simulink model "MVDR_example_hdl_4x4_systolic"  (R2020a)
settings: Solver=FixedStepDiscrete  StartTime=0.0  StopTime=stoptime  RelTol=1e-3
InitFcn:
  | model_init
values from neighbouring files (symbols this model uses):
  BackSubstitutePrototype = fi(0, matrixdivbacksub_dt)    [model_init.m]
  matrixDivDelay = NumberOfCORDICIterations*10 + 86    [model_init.m]
  movavg_bitshift = nextpow2(sqrt(windowSize))    [model_init.m]
  mvdrPipelineDelay = covMatDelay+movAvgDelay+matrixDivDelay+normResponseDelay    [model_init.m]
  numArrayElements = 4    [model_init.m]
  NumberOfCORDICIterations = matrixdivin_dt.WordLength - 1    [model_init.m]
  srcAngles = [20 60]    [model_init.m]
  sv = step(steeringVector,fc,[scanAngle; 0])    [model_init.m]
  Ts = 1/fs    (= 7.8125e-09)    [model_init.m]
  windowSize = 1024    [model_init.m]
libraries: hdlsllib x249, simulink x44, commfilt2 x4, commrfcorlib x3, commsync2 x3, commrflib2 x2, commrandsrc3 x2, phasedtxrxlib x2, commdigbbndcpm2 x1, dspsolvers x1, embreciprocals x1, commdigbbndpm3 x1
(part 3 of 11)

== system MVDR_example_hdl_4x4_systolic/MVDR HDL/Compute Weight Vector/Matrix Left Divide/CORDIC/4x4 Complex CORDIC Matrix Left Divide/Q'B, R 4x4 Complex CORDIC Systolic Array/Complex Row Rotation with real pivots ==
  note: The pivots are real, so you don't need to
      | rotate the first elements to real, but you do
      | need to account for the delay in the parallel
      | elements that are rotating their first elements
      | to real.
  x : Inport
  y : Inport  Port=2
  u : Inport  Port=3
  v : Inport  Port=4
  validIn : Inport  Port=5
  validIn from rotate first element to real : Inport  Port=6
  Delay17 : Delay  DelayLength=1
  Delay18 : Delay  DelayLength=1
  Delay2 : Delay  DelayLength=1
  Inverse CORDIC Gain1 : Subsystem  TreatAsAtomicUnit=on  mask{NumberOfCORDICIterations=NumberOfCORDICIterations}
      mask prompts: NumberOfCORDICIterations "Number of CORDIC Iterations"
      mask Display: disp('1/An')
  Inverse CORDIC Gain2 : Subsystem  TreatAsAtomicUnit=on  mask{NumberOfCORDICIterations=NumberOfCORDICIterations}
      mask prompts: NumberOfCORDICIterations "Number of CORDIC Iterations"
      mask Display: disp('1/An')
  Inverse CORDIC Gain3 : Subsystem  TreatAsAtomicUnit=on  mask{NumberOfCORDICIterations=NumberOfCORDICIterations}
      mask prompts: NumberOfCORDICIterations "Number of CORDIC Iterations"
      mask Display: disp('1/An')
  Inverse CORDIC Gain4 : Subsystem  TreatAsAtomicUnit=on  mask{NumberOfCORDICIterations=NumberOfCORDICIterations}
      mask prompts: NumberOfCORDICIterations "Number of CORDIC Iterations"
      mask Display: disp('1/An')
  "Q'B, R Row Rotations - Complex" : Subsystem  TreatAsAtomicUnit=on  mask{NumberOfCORDICIterations=NumberOfCORDICIterations}
      mask prompts: NumberOfCORDICIterations "Number of CORDIC Iterations"
  QR 3rd and 4th Quadrant Compensation : MATLAB Function  TreatAsAtomicUnit=on
  Unit Delay Enabled Synchronous{,1..7,9..12} (12 alike) : hdlsllib/Discrete/Unit Delay Enabled Synchronous  InitialCondition=0.0  SampleTime=-1
      settings: SourceProductBaseCode=SL
  ValidIn to Ready Logic : Subsystem
  ValidIn to Ready Logic1 : Subsystem
  y = u(2:end) : MATLAB Function  TreatAsAtomicUnit=on
  x' : Outport  VectorParamsAs1DForOutWhenUnconnected=off
  y' : Outport  Port=2  VectorParamsAs1DForOutWhenUnconnected=off
  u' : Outport  Port=3  VectorParamsAs1DForOutWhenUnconnected=off
  v' : Outport  Port=4  VectorParamsAs1DForOutWhenUnconnected=off
  validOut : Outport  Port=5  VectorParamsAs1DForOutWhenUnconnected=off
  ready : Outport  Port=6  VectorParamsAs1DForOutWhenUnconnected=off
  wires:
  Inverse CORDIC Gain3/1(Out1) -> Unit Delay Enabled Synchronous4/1
  Inverse CORDIC Gain4/1(Out1) -> Unit Delay Enabled Synchronous7/1
  x/1 -> Unit Delay Enabled Synchronous3/1
  Unit Delay Enabled Synchronous3/1 -> Unit Delay Enabled Synchronous12/1
  y/1 -> Unit Delay Enabled Synchronous2/1
  u/1 -> Unit Delay Enabled Synchronous1/1
  Unit Delay Enabled Synchronous1/1 -> Unit Delay Enabled Synchronous10/1
  v/1 -> Unit Delay Enabled Synchronous/1
  Inverse CORDIC Gain2/1(Out1) -> Unit Delay Enabled Synchronous5/1
  "Q'B, R Row Rotations - Complex"/1(x_out) -> Inverse CORDIC Gain4/1(In1)
  "Q'B, R Row Rotations - Complex"/3(u_out) -> Inverse CORDIC Gain2/1(In1)
  "Q'B, R Row Rotations - Complex"/4(v_out) -> Inverse CORDIC Gain3/1(In1)
  Inverse CORDIC Gain1/1(Out1) -> Unit Delay Enabled Synchronous6/1
  y = u(2:end)/1(y) -> y'/1
  Unit Delay Enabled Synchronous2/1 -> Unit Delay Enabled Synchronous11/1
  Unit Delay Enabled Synchronous/1 -> Unit Delay Enabled Synchronous9/1
  "Q'B, R Row Rotations - Complex"/2(y_out) -> Inverse CORDIC Gain1/1(In1)
  Unit Delay Enabled Synchronous7/1 -> x'/1
  Unit Delay Enabled Synchronous6/1 -> y = u(2:end)/1(u)
  Unit Delay Enabled Synchronous5/1 -> u'/1
  Unit Delay Enabled Synchronous4/1 -> v'/1
  validIn from rotate first element to real/1 -> ValidIn to Ready Logic1/2(validIn), Delay2/1, Unit Delay Enabled Synchronous9/2, Unit Delay Enabled Synchronous10/2, Unit Delay Enabled Synchronous11/2, Unit Delay Enabled Synchronous12/2
  Delay17/1 -> validOut/1
  Delay18/1 -> ready/1
  "Q'B, R Row Rotations - Complex"/5(validOut) -> Delay17/1, Unit Delay Enabled Synchronous4/2, Unit Delay Enabled Synchronous5/2, Unit Delay Enabled Synchronous6/2, Unit Delay Enabled Synchronous7/2
  validIn/1 -> Unit Delay Enabled Synchronous/2, Unit Delay Enabled Synchronous1/2, Unit Delay Enabled Synchronous2/2, Unit Delay Enabled Synchronous3/2
  Unit Delay Enabled Synchronous12/1 -> QR 3rd and 4th Quadrant Compensation/1(x)
  Unit Delay Enabled Synchronous11/1 -> QR 3rd and 4th Quadrant Compensation/2(y)
  Unit Delay Enabled Synchronous10/1 -> QR 3rd and 4th Quadrant Compensation/3(u)
  Unit Delay Enabled Synchronous9/1 -> QR 3rd and 4th Quadrant Compensation/4(v)
  ValidIn to Ready Logic/1(readyOut) -> ValidIn to Ready Logic1/1(readyIn)
  ValidIn to Ready Logic1/1(readyOut) -> Delay18/1
  QR 3rd and 4th Quadrant Compensation/1(x_out) -> "Q'B, R Row Rotations - Complex"/1(x)
  QR 3rd and 4th Quadrant Compensation/2(y_out) -> "Q'B, R Row Rotations - Complex"/2(y)
  QR 3rd and 4th Quadrant Compensation/3(u_out) -> "Q'B, R Row Rotations - Complex"/3(u)
  QR 3rd and 4th Quadrant Compensation/4(v_out) -> "Q'B, R Row Rotations - Complex"/4(v)
  Delay2/1 -> "Q'B, R Row Rotations - Complex"/5(validIn), ValidIn to Ready Logic/2(validIn)
  "Q'B, R Row Rotations - Complex"/6(ready) -> ValidIn to Ready Logic/1(readyIn)

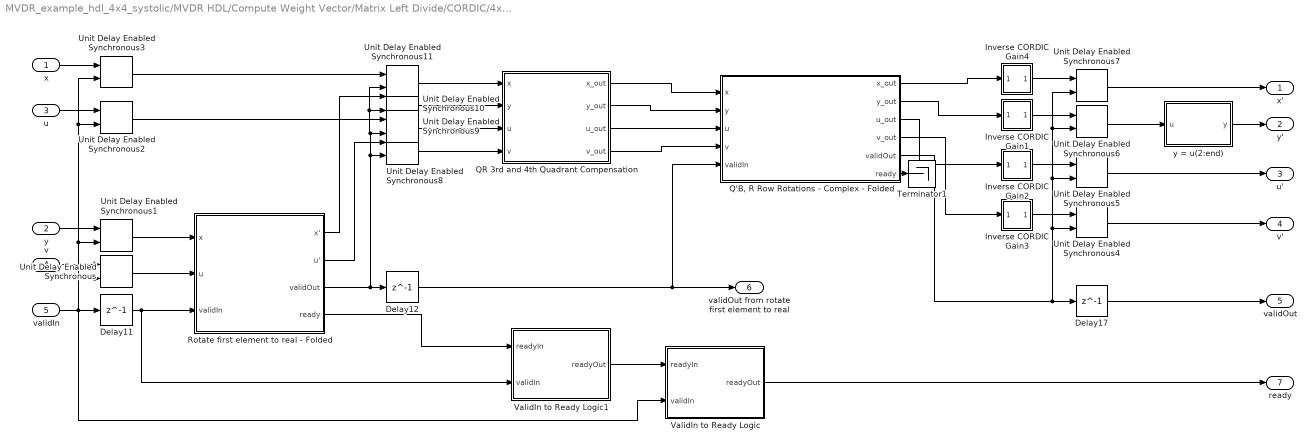
== system MVDR_example_hdl_4x4_systolic/MVDR HDL/Compute Weight Vector/Matrix Left Divide/CORDIC/4x4 Complex CORDIC Matrix Left Divide/Q'B, R 4x4 Complex CORDIC Systolic Array/Complex Row Rotation 1 ==
  x : Inport
  y : Inport  Port=2
  u : Inport  Port=3
  v : Inport  Port=4
  validIn : Inport  Port=5
  Delay11 : Delay  DelayLength=1
  Delay12 : Delay  DelayLength=1
  Delay17 : Delay  DelayLength=1
  Inverse CORDIC Gain1 : Subsystem  TreatAsAtomicUnit=on  mask{NumberOfCORDICIterations=NumberOfCORDICIterations}
      mask prompts: NumberOfCORDICIterations "Number of CORDIC Iterations"
      mask Display: disp('1/An')
  Inverse CORDIC Gain2 : Subsystem  TreatAsAtomicUnit=on  mask{NumberOfCORDICIterations=NumberOfCORDICIterations}
      mask prompts: NumberOfCORDICIterations "Number of CORDIC Iterations"
      mask Display: disp('1/An')
  Inverse CORDIC Gain3 : Subsystem  TreatAsAtomicUnit=on  mask{NumberOfCORDICIterations=NumberOfCORDICIterations}
      mask prompts: NumberOfCORDICIterations "Number of CORDIC Iterations"
      mask Display: disp('1/An')
  Inverse CORDIC Gain4 : Subsystem  TreatAsAtomicUnit=on  mask{NumberOfCORDICIterations=NumberOfCORDICIterations}
      mask prompts: NumberOfCORDICIterations "Number of CORDIC Iterations"
      mask Display: disp('1/An')
  "Q'B, R Row Rotations - Complex - Folded" : Subsystem  TreatAsAtomicUnit=on  mask{NumberOfCORDICIterations=NumberOfCORDICIterations}
      mask prompts: NumberOfCORDICIterations "Number of CORDIC Iterations"
  QR 3rd and 4th Quadrant Compensation : MATLAB Function  TreatAsAtomicUnit=on
  Rotate first element to real - Folded : Subsystem  TreatAsAtomicUnit=on  mask{NumberOfCORDICIterations=NumberOfCORDICIterations}
      mask prompts: NumberOfCORDICIterations "Number of CORDIC Iterations"
  Terminator1 : Terminator
  Unit Delay Enabled Synchronous{,1..11} (12 alike) : hdlsllib/Discrete/Unit Delay Enabled Synchronous  InitialCondition=0.0  SampleTime=-1
      settings: SourceProductBaseCode=SL
  ValidIn to Ready Logic : Subsystem
  ValidIn to Ready Logic1 : Subsystem
  y = u(2:end) : MATLAB Function  TreatAsAtomicUnit=on
  x' : Outport  VectorParamsAs1DForOutWhenUnconnected=off
  y' : Outport  Port=2  VectorParamsAs1DForOutWhenUnconnected=off
  u' : Outport  Port=3  VectorParamsAs1DForOutWhenUnconnected=off
  v' : Outport  Port=4  VectorParamsAs1DForOutWhenUnconnected=off
  validOut : Outport  Port=5  VectorParamsAs1DForOutWhenUnconnected=off
  validOut from rotate first element to real : Outport  Port=6  VectorParamsAs1DForOutWhenUnconnected=off
  ready : Outport  Port=7  VectorParamsAs1DForOutWhenUnconnected=off
  wires:
  "Q'B, R Row Rotations - Complex - Folded"/2(y_out) -> Inverse CORDIC Gain1/1(In1)
  "Q'B, R Row Rotations - Complex - Folded"/4(v_out) -> Inverse CORDIC Gain3/1(In1)
  "Q'B, R Row Rotations - Complex - Folded"/3(u_out) -> Inverse CORDIC Gain2/1(In1)
  ValidIn to Ready Logic/1(readyOut) -> ready/1
  x/1 -> Unit Delay Enabled Synchronous3/1
  ValidIn to Ready Logic1/1(readyOut) -> ValidIn to Ready Logic/1(readyIn)
  Inverse CORDIC Gain1/1(Out1) -> Unit Delay Enabled Synchronous6/1
  Unit Delay Enabled Synchronous4/1 -> v'/1
  Unit Delay Enabled Synchronous3/1 -> Unit Delay Enabled Synchronous11/1
  Rotate first element to real - Folded/4(ready) -> ValidIn to Ready Logic1/1(readyIn)
  Delay17/1 -> validOut/1
  Inverse CORDIC Gain2/1(Out1) -> Unit Delay Enabled Synchronous5/1
  Unit Delay Enabled Synchronous7/1 -> x'/1
  Delay12/1 -> validOut from rotate first element to real/1, "Q'B, R Row Rotations - Complex - Folded"/5(validIn)
  validIn/1 -> ValidIn to Ready Logic/2(validIn), Unit Delay Enabled Synchronous/2, Unit Delay Enabled Synchronous1/2, Unit Delay Enabled Synchronous2/2, Unit Delay Enabled Synchronous3/2, Delay11/1
  "Q'B, R Row Rotations - Complex - Folded"/6(ready) -> Terminator1/1
  v/1 -> Unit Delay Enabled Synchronous/1
  y/1 -> Unit Delay Enabled Synchronous1/1
  Unit Delay Enabled Synchronous5/1 -> u'/1
  "Q'B, R Row Rotations - Complex - Folded"/5(validOut) -> Delay17/1, Unit Delay Enabled Synchronous4/2, Unit Delay Enabled Synchronous5/2, Unit Delay Enabled Synchronous6/2, Unit Delay Enabled Synchronous7/2
  u/1 -> Unit Delay Enabled Synchronous2/1
  Unit Delay Enabled Synchronous6/1 -> y = u(2:end)/1(u)
  Inverse CORDIC Gain3/1(Out1) -> Unit Delay Enabled Synchronous4/1
  Unit Delay Enabled Synchronous2/1 -> Unit Delay Enabled Synchronous9/1
  Inverse CORDIC Gain4/1(Out1) -> Unit Delay Enabled Synchronous7/1
  "Q'B, R Row Rotations - Complex - Folded"/1(x_out) -> Inverse CORDIC Gain4/1(In1)
  Unit Delay Enabled Synchronous/1 -> Rotate first element to real - Folded/2(u)
  y = u(2:end)/1(y) -> y'/1
  Unit Delay Enabled Synchronous1/1 -> Rotate first element to real - Folded/1(x)
  Rotate first element to real - Folded/3(validOut) -> Unit Delay Enabled Synchronous10/2, Unit Delay Enabled Synchronous11/2, Unit Delay Enabled Synchronous9/2, Unit Delay Enabled Synchronous8/2, Delay12/1
  Delay11/1 -> ValidIn to Ready Logic1/2(validIn), Rotate first element to real - Folded/3(validIn)
  Rotate first element to real - Folded/1(x') -> Unit Delay Enabled Synchronous10/1
  Unit Delay Enabled Synchronous10/1 -> QR 3rd and 4th Quadrant Compensation/2(y)
  Rotate first element to real - Folded/2(u') -> Unit Delay Enabled Synchronous8/1
  Unit Delay Enabled Synchronous8/1 -> QR 3rd and 4th Quadrant Compensation/4(v)
  Unit Delay Enabled Synchronous11/1 -> QR 3rd and 4th Quadrant Compensation/1(x)
  Unit Delay Enabled Synchronous9/1 -> QR 3rd and 4th Quadrant Compensation/3(u)
  QR 3rd and 4th Quadrant Compensation/3(u_out) -> "Q'B, R Row Rotations - Complex - Folded"/3(u)
  QR 3rd and 4th Quadrant Compensation/2(y_out) -> "Q'B, R Row Rotations - Complex - Folded"/2(y)
  QR 3rd and 4th Quadrant Compensation/4(v_out) -> "Q'B, R Row Rotations - Complex - Folded"/4(v)
  QR 3rd and 4th Quadrant Compensation/1(x_out) -> "Q'B, R Row Rotations - Complex - Folded"/1(x)

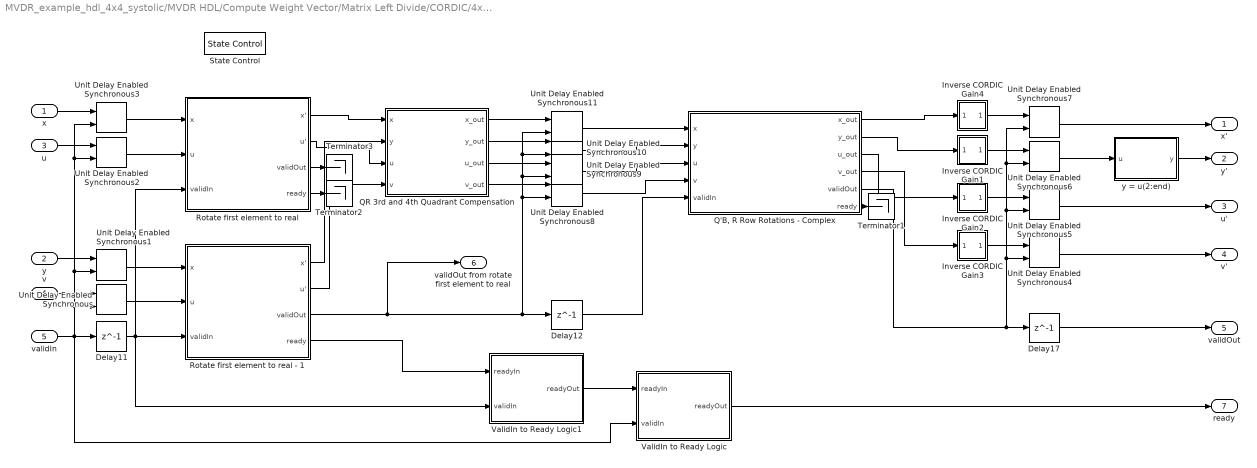
== system MVDR_example_hdl_4x4_systolic/MVDR HDL/Compute Weight Vector/Matrix Left Divide/CORDIC/4x4 Complex CORDIC Matrix Left Divide/Q'B, R 4x4 Complex CORDIC Systolic Array/Leading Complex Row Rotation ==
  x : Inport
  y : Inport  Port=2
  u : Inport  Port=3
  v : Inport  Port=4
  validIn : Inport  Port=5
  Delay11 : Delay  DelayLength=1
  Delay12 : Delay  DelayLength=1
  Delay17 : Delay  DelayLength=1
  Inverse CORDIC Gain1 : Subsystem  TreatAsAtomicUnit=on  mask{NumberOfCORDICIterations=NumberOfCORDICIterations}
      mask prompts: NumberOfCORDICIterations "Number of CORDIC Iterations"
      mask Display: disp('1/An')
  Inverse CORDIC Gain2 : Subsystem  TreatAsAtomicUnit=on  mask{NumberOfCORDICIterations=NumberOfCORDICIterations}
      mask prompts: NumberOfCORDICIterations "Number of CORDIC Iterations"
      mask Display: disp('1/An')
  Inverse CORDIC Gain3 : Subsystem  TreatAsAtomicUnit=on  mask{NumberOfCORDICIterations=NumberOfCORDICIterations}
      mask prompts: NumberOfCORDICIterations "Number of CORDIC Iterations"
      mask Display: disp('1/An')
  Inverse CORDIC Gain4 : Subsystem  TreatAsAtomicUnit=on  mask{NumberOfCORDICIterations=NumberOfCORDICIterations}
      mask prompts: NumberOfCORDICIterations "Number of CORDIC Iterations"
      mask Display: disp('1/An')
  "Q'B, R Row Rotations - Complex" : Subsystem  TreatAsAtomicUnit=on  mask{NumberOfCORDICIterations=NumberOfCORDICIterations}
      mask prompts: NumberOfCORDICIterations "Number of CORDIC Iterations"
  QR 3rd and 4th Quadrant Compensation : MATLAB Function  TreatAsAtomicUnit=on
  Rotate first element to real : Subsystem  TreatAsAtomicUnit=on  mask{NumberOfCORDICIterations=NumberOfCORDICIterations}
      mask prompts: NumberOfCORDICIterations "Number of CORDIC Iterations"
  Rotate first element to real - 1 : Subsystem  TreatAsAtomicUnit=on  mask{NumberOfCORDICIterations=NumberOfCORDICIterations}
      mask prompts: NumberOfCORDICIterations "Number of CORDIC Iterations"
  State Control : StateControl  StateControl=Synchronous
  Terminator1 : Terminator
  Terminator2 : Terminator
  Terminator3 : Terminator
  Unit Delay Enabled Synchronous{,1..11} (12 alike) : hdlsllib/Discrete/Unit Delay Enabled Synchronous  InitialCondition=0.0  SampleTime=-1
      settings: SourceProductBaseCode=SL
  ValidIn to Ready Logic : Subsystem
  ValidIn to Ready Logic1 : Subsystem
  y = u(2:end) : MATLAB Function  TreatAsAtomicUnit=on
  x' : Outport  VectorParamsAs1DForOutWhenUnconnected=off
  y' : Outport  Port=2  VectorParamsAs1DForOutWhenUnconnected=off
  u' : Outport  Port=3  VectorParamsAs1DForOutWhenUnconnected=off
  v' : Outport  Port=4  VectorParamsAs1DForOutWhenUnconnected=off
  validOut : Outport  Port=5  VectorParamsAs1DForOutWhenUnconnected=off
  validOut from rotate first element to real : Outport  Port=6  VectorParamsAs1DForOutWhenUnconnected=off
  ready : Outport  Port=7  VectorParamsAs1DForOutWhenUnconnected=off
  wires:
  QR 3rd and 4th Quadrant Compensation/1(x_out) -> Unit Delay Enabled Synchronous11/1
  QR 3rd and 4th Quadrant Compensation/3(u_out) -> Unit Delay Enabled Synchronous9/1
  QR 3rd and 4th Quadrant Compensation/2(y_out) -> Unit Delay Enabled Synchronous10/1
  QR 3rd and 4th Quadrant Compensation/4(v_out) -> Unit Delay Enabled Synchronous8/1
  Inverse CORDIC Gain3/1(Out1) -> Unit Delay Enabled Synchronous4/1
  Inverse CORDIC Gain4/1(Out1) -> Unit Delay Enabled Synchronous7/1
  x/1 -> Unit Delay Enabled Synchronous3/1
  Unit Delay Enabled Synchronous3/1 -> Rotate first element to real/1(x)
  u/1 -> Unit Delay Enabled Synchronous2/1
  v/1 -> Unit Delay Enabled Synchronous/1
  Inverse CORDIC Gain2/1(Out1) -> Unit Delay Enabled Synchronous5/1
  Unit Delay Enabled Synchronous11/1 -> "Q'B, R Row Rotations - Complex"/1(x)
  Unit Delay Enabled Synchronous10/1 -> "Q'B, R Row Rotations - Complex"/2(y)
  Unit Delay Enabled Synchronous9/1 -> "Q'B, R Row Rotations - Complex"/3(u)
  Unit Delay Enabled Synchronous8/1 -> "Q'B, R Row Rotations - Complex"/4(v)
  "Q'B, R Row Rotations - Complex"/1(x_out) -> Inverse CORDIC Gain4/1(In1)
  "Q'B, R Row Rotations - Complex"/3(u_out) -> Inverse CORDIC Gain2/1(In1)
  "Q'B, R Row Rotations - Complex"/4(v_out) -> Inverse CORDIC Gain3/1(In1)
  Inverse CORDIC Gain1/1(Out1) -> Unit Delay Enabled Synchronous6/1
  y = u(2:end)/1(y) -> y'/1
  Unit Delay Enabled Synchronous1/1 -> Rotate first element to real - 1/1(x)
  Unit Delay Enabled Synchronous/1 -> Rotate first element to real - 1/2(u)
  Rotate first element to real - 1/1(x') -> QR 3rd and 4th Quadrant Compensation/2(y)
  Rotate first element to real - 1/2(u') -> QR 3rd and 4th Quadrant Compensation/4(v)
  "Q'B, R Row Rotations - Complex"/2(y_out) -> Inverse CORDIC Gain1/1(In1)
  validIn/1 -> ValidIn to Ready Logic/2(validIn), Unit Delay Enabled Synchronous/2, Unit Delay Enabled Synchronous1/2, Unit Delay Enabled Synchronous2/2, Unit Delay Enabled Synchronous3/2, Delay11/1
  Delay11/1 -> ValidIn to Ready Logic1/2(validIn), Rotate first element to real/3(validIn), Rotate first element to real - 1/3(validIn)
  Rotate first element to real - 1/3(validOut) -> Unit Delay Enabled Synchronous8/2, Unit Delay Enabled Synchronous9/2, Unit Delay Enabled Synchronous10/2, Unit Delay Enabled Synchronous11/2, Delay12/1, validOut from rotate first element to real/1
  Unit Delay Enabled Synchronous7/1 -> x'/1
  Unit Delay Enabled Synchronous6/1 -> y = u(2:end)/1(u)
  Unit Delay Enabled Synchronous5/1 -> u'/1
  Unit Delay Enabled Synchronous4/1 -> v'/1
  Delay12/1 -> "Q'B, R Row Rotations - Complex"/5(validIn)
  "Q'B, R Row Rotations - Complex"/5(validOut) -> Delay17/1, Unit Delay Enabled Synchronous4/2, Unit Delay Enabled Synchronous5/2, Unit Delay Enabled Synchronous6/2, Unit Delay Enabled Synchronous7/2
  Delay17/1 -> validOut/1
  Rotate first element to real/4(ready) -> Terminator2/1
  Rotate first element to real/3(validOut) -> Terminator3/1
  Rotate first element to real/1(x') -> QR 3rd and 4th Quadrant Compensation/1(x)
  Rotate first element to real/2(u') -> QR 3rd and 4th Quadrant Compensation/3(u)
  Unit Delay Enabled Synchronous2/1 -> Rotate first element to real/2(u)
  y/1 -> Unit Delay Enabled Synchronous1/1
  ValidIn to Ready Logic/1(readyOut) -> ready/1
  ValidIn to Ready Logic1/1(readyOut) -> ValidIn to Ready Logic/1(readyIn)
  "Q'B, R Row Rotations - Complex"/6(ready) -> Terminator1/1
  Rotate first element to real - 1/4(ready) -> ValidIn to Ready Logic1/1(readyIn)

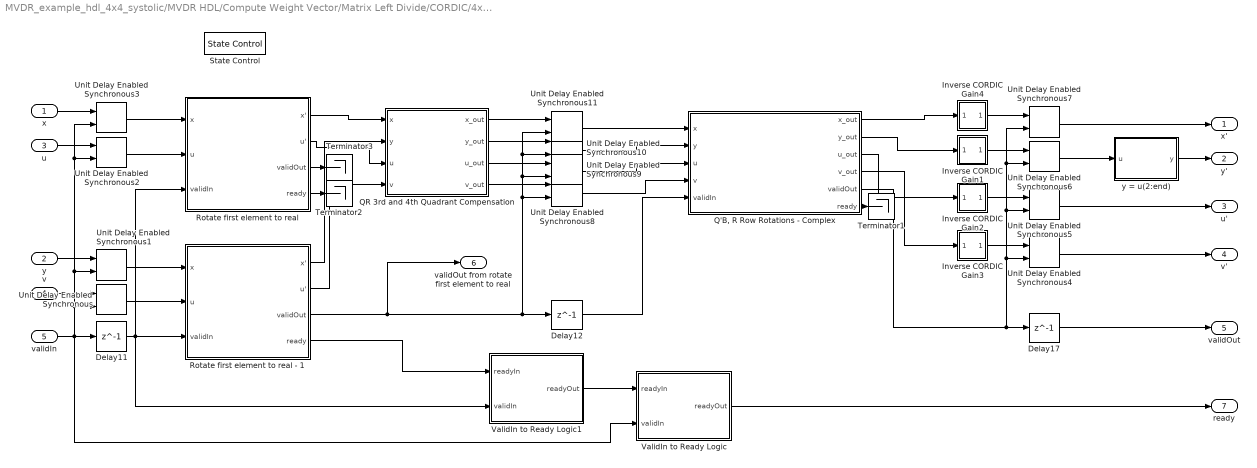
== system MVDR_example_hdl_4x4_systolic/MVDR HDL/Compute Weight Vector/Matrix Left Divide/CORDIC/4x4 Complex CORDIC Matrix Left Divide/Q'B, R 4x4 Complex CORDIC Systolic Array/Leading Complex Row Rotation - 2 ==
  x : Inport
  y : Inport  Port=2
  u : Inport  Port=3
  v : Inport  Port=4
  validIn : Inport  Port=5
  Delay11 : Delay  DelayLength=1
  Delay12 : Delay  DelayLength=1
  Delay17 : Delay  DelayLength=1
  Inverse CORDIC Gain1 : Subsystem  TreatAsAtomicUnit=on  mask{NumberOfCORDICIterations=NumberOfCORDICIterations}
      mask prompts: NumberOfCORDICIterations "Number of CORDIC Iterations"
      mask Display: disp('1/An')
  Inverse CORDIC Gain2 : Subsystem  TreatAsAtomicUnit=on  mask{NumberOfCORDICIterations=NumberOfCORDICIterations}
      mask prompts: NumberOfCORDICIterations "Number of CORDIC Iterations"
      mask Display: disp('1/An')
  Inverse CORDIC Gain3 : Subsystem  TreatAsAtomicUnit=on  mask{NumberOfCORDICIterations=NumberOfCORDICIterations}
      mask prompts: NumberOfCORDICIterations "Number of CORDIC Iterations"
      mask Display: disp('1/An')
  Inverse CORDIC Gain4 : Subsystem  TreatAsAtomicUnit=on  mask{NumberOfCORDICIterations=NumberOfCORDICIterations}
      mask prompts: NumberOfCORDICIterations "Number of CORDIC Iterations"
      mask Display: disp('1/An')
  "Q'B, R Row Rotations - Complex" : Subsystem  TreatAsAtomicUnit=on  mask{NumberOfCORDICIterations=NumberOfCORDICIterations}
      mask prompts: NumberOfCORDICIterations "Number of CORDIC Iterations"
  QR 3rd and 4th Quadrant Compensation : MATLAB Function  TreatAsAtomicUnit=on
  Rotate first element to real : Subsystem  TreatAsAtomicUnit=on  mask{NumberOfCORDICIterations=NumberOfCORDICIterations}
      mask prompts: NumberOfCORDICIterations "Number of CORDIC Iterations"
  Rotate first element to real - 1 : Subsystem  TreatAsAtomicUnit=on  mask{NumberOfCORDICIterations=NumberOfCORDICIterations}
      mask prompts: NumberOfCORDICIterations "Number of CORDIC Iterations"
  State Control : StateControl  StateControl=Synchronous
  Terminator1 : Terminator
  Terminator2 : Terminator
  Terminator3 : Terminator
  Unit Delay Enabled Synchronous{,1..11} (12 alike) : hdlsllib/Discrete/Unit Delay Enabled Synchronous  InitialCondition=0.0  SampleTime=-1
      settings: SourceProductBaseCode=SL
  ValidIn to Ready Logic : Subsystem
  ValidIn to Ready Logic1 : Subsystem
  y = u(2:end) : MATLAB Function  TreatAsAtomicUnit=on
  x' : Outport  VectorParamsAs1DForOutWhenUnconnected=off
  y' : Outport  Port=2  VectorParamsAs1DForOutWhenUnconnected=off
  u' : Outport  Port=3  VectorParamsAs1DForOutWhenUnconnected=off
  v' : Outport  Port=4  VectorParamsAs1DForOutWhenUnconnected=off
  validOut : Outport  Port=5  VectorParamsAs1DForOutWhenUnconnected=off
  validOut from rotate first element to real : Outport  Port=6  VectorParamsAs1DForOutWhenUnconnected=off
  ready : Outport  Port=7  VectorParamsAs1DForOutWhenUnconnected=off
  wires:
  Rotate first element to real - 1/4(ready) -> ValidIn to Ready Logic1/1(readyIn)
  "Q'B, R Row Rotations - Complex"/6(ready) -> Terminator1/1
  ValidIn to Ready Logic1/1(readyOut) -> ValidIn to Ready Logic/1(readyIn)
  ValidIn to Ready Logic/1(readyOut) -> ready/1
  y/1 -> Unit Delay Enabled Synchronous1/1
  Unit Delay Enabled Synchronous2/1 -> Rotate first element to real/2(u)
  Rotate first element to real/2(u') -> QR 3rd and 4th Quadrant Compensation/3(u)
  Rotate first element to real/1(x') -> QR 3rd and 4th Quadrant Compensation/1(x)
  Rotate first element to real/3(validOut) -> Terminator3/1
  Rotate first element to real/4(ready) -> Terminator2/1
  Delay17/1 -> validOut/1
  "Q'B, R Row Rotations - Complex"/5(validOut) -> Unit Delay Enabled Synchronous7/2, Unit Delay Enabled Synchronous6/2, Unit Delay Enabled Synchronous5/2, Unit Delay Enabled Synchronous4/2, Delay17/1
  Delay12/1 -> "Q'B, R Row Rotations - Complex"/5(validIn)
  Unit Delay Enabled Synchronous4/1 -> v'/1
  Unit Delay Enabled Synchronous5/1 -> u'/1
  Unit Delay Enabled Synchronous6/1 -> y = u(2:end)/1(u)
  Unit Delay Enabled Synchronous7/1 -> x'/1
  Rotate first element to real - 1/3(validOut) -> validOut from rotate first element to real/1, Delay12/1, Unit Delay Enabled Synchronous11/2, Unit Delay Enabled Synchronous10/2, Unit Delay Enabled Synchronous9/2, Unit Delay Enabled Synchronous8/2
  Delay11/1 -> Rotate first element to real - 1/3(validIn), Rotate first element to real/3(validIn), ValidIn to Ready Logic1/2(validIn)
  validIn/1 -> Delay11/1, Unit Delay Enabled Synchronous3/2, Unit Delay Enabled Synchronous2/2, Unit Delay Enabled Synchronous1/2, Unit Delay Enabled Synchronous/2, ValidIn to Ready Logic/2(validIn)
  "Q'B, R Row Rotations - Complex"/2(y_out) -> Inverse CORDIC Gain1/1(In1)
  Rotate first element to real - 1/2(u') -> QR 3rd and 4th Quadrant Compensation/4(v)
  Rotate first element to real - 1/1(x') -> QR 3rd and 4th Quadrant Compensation/2(y)
  Unit Delay Enabled Synchronous/1 -> Rotate first element to real - 1/2(u)
  Unit Delay Enabled Synchronous1/1 -> Rotate first element to real - 1/1(x)
  y = u(2:end)/1(y) -> y'/1
  Inverse CORDIC Gain1/1(Out1) -> Unit Delay Enabled Synchronous6/1
  "Q'B, R Row Rotations - Complex"/4(v_out) -> Inverse CORDIC Gain3/1(In1)
  "Q'B, R Row Rotations - Complex"/3(u_out) -> Inverse CORDIC Gain2/1(In1)
  "Q'B, R Row Rotations - Complex"/1(x_out) -> Inverse CORDIC Gain4/1(In1)
  Unit Delay Enabled Synchronous8/1 -> "Q'B, R Row Rotations - Complex"/4(v)
  Unit Delay Enabled Synchronous9/1 -> "Q'B, R Row Rotations - Complex"/3(u)
  Unit Delay Enabled Synchronous10/1 -> "Q'B, R Row Rotations - Complex"/2(y)
  Unit Delay Enabled Synchronous11/1 -> "Q'B, R Row Rotations - Complex"/1(x)
  Inverse CORDIC Gain2/1(Out1) -> Unit Delay Enabled Synchronous5/1
  v/1 -> Unit Delay Enabled Synchronous/1
  u/1 -> Unit Delay Enabled Synchronous2/1
  Unit Delay Enabled Synchronous3/1 -> Rotate first element to real/1(x)
  x/1 -> Unit Delay Enabled Synchronous3/1
  Inverse CORDIC Gain4/1(Out1) -> Unit Delay Enabled Synchronous7/1
  Inverse CORDIC Gain3/1(Out1) -> Unit Delay Enabled Synchronous4/1
  QR 3rd and 4th Quadrant Compensation/4(v_out) -> Unit Delay Enabled Synchronous8/1
  QR 3rd and 4th Quadrant Compensation/2(y_out) -> Unit Delay Enabled Synchronous10/1
  QR 3rd and 4th Quadrant Compensation/3(u_out) -> Unit Delay Enabled Synchronous9/1
  QR 3rd and 4th Quadrant Compensation/1(x_out) -> Unit Delay Enabled Synchronous11/1

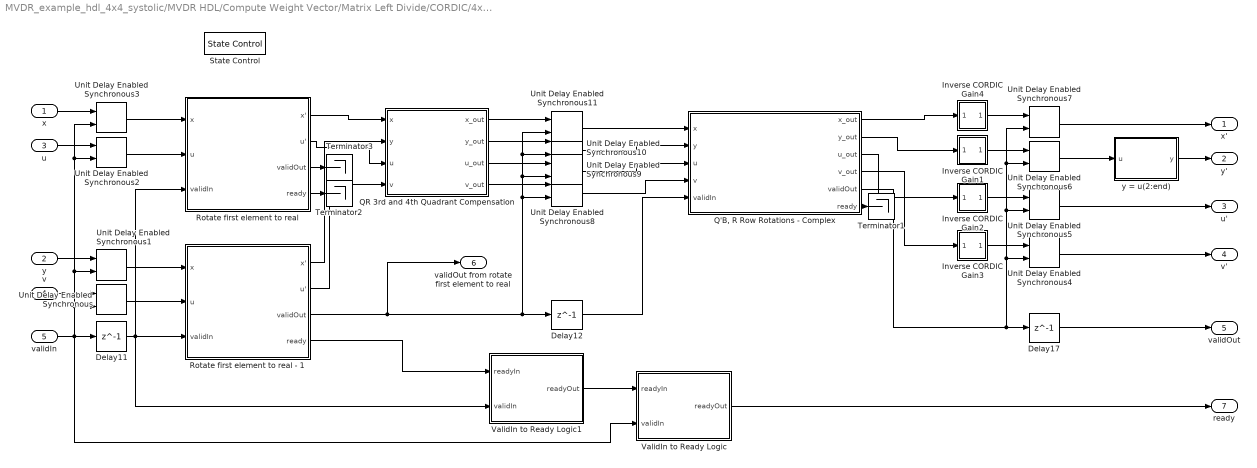
== system MVDR_example_hdl_4x4_systolic/MVDR HDL/Compute Weight Vector/Matrix Left Divide/CORDIC/4x4 Complex CORDIC Matrix Left Divide/Q'B, R 4x4 Complex CORDIC Systolic Array/Leading Complex Row Rotation - 3 ==
  x : Inport
  y : Inport  Port=2
  u : Inport  Port=3
  v : Inport  Port=4
  validIn : Inport  Port=5
  Delay11 : Delay  DelayLength=1
  Delay12 : Delay  DelayLength=1
  Delay17 : Delay  DelayLength=1
  Inverse CORDIC Gain1 : Subsystem  TreatAsAtomicUnit=on  mask{NumberOfCORDICIterations=NumberOfCORDICIterations}
      mask prompts: NumberOfCORDICIterations "Number of CORDIC Iterations"
      mask Display: disp('1/An')
  Inverse CORDIC Gain2 : Subsystem  TreatAsAtomicUnit=on  mask{NumberOfCORDICIterations=NumberOfCORDICIterations}
      mask prompts: NumberOfCORDICIterations "Number of CORDIC Iterations"
      mask Display: disp('1/An')
  Inverse CORDIC Gain3 : Subsystem  TreatAsAtomicUnit=on  mask{NumberOfCORDICIterations=NumberOfCORDICIterations}
      mask prompts: NumberOfCORDICIterations "Number of CORDIC Iterations"
      mask Display: disp('1/An')
  Inverse CORDIC Gain4 : Subsystem  TreatAsAtomicUnit=on  mask{NumberOfCORDICIterations=NumberOfCORDICIterations}
      mask prompts: NumberOfCORDICIterations "Number of CORDIC Iterations"
      mask Display: disp('1/An')
  "Q'B, R Row Rotations - Complex" : Subsystem  TreatAsAtomicUnit=on  mask{NumberOfCORDICIterations=NumberOfCORDICIterations}
      mask prompts: NumberOfCORDICIterations "Number of CORDIC Iterations"
  QR 3rd and 4th Quadrant Compensation : MATLAB Function  TreatAsAtomicUnit=on
  Rotate first element to real : Subsystem  TreatAsAtomicUnit=on  mask{NumberOfCORDICIterations=NumberOfCORDICIterations}
      mask prompts: NumberOfCORDICIterations "Number of CORDIC Iterations"
  Rotate first element to real - 1 : Subsystem  TreatAsAtomicUnit=on  mask{NumberOfCORDICIterations=NumberOfCORDICIterations}
      mask prompts: NumberOfCORDICIterations "Number of CORDIC Iterations"
  State Control : StateControl  StateControl=Synchronous
  Terminator1 : Terminator
  Terminator2 : Terminator
  Terminator3 : Terminator
  Unit Delay Enabled Synchronous{,1..11} (12 alike) : hdlsllib/Discrete/Unit Delay Enabled Synchronous  InitialCondition=0.0  SampleTime=-1
      settings: SourceProductBaseCode=SL
  ValidIn to Ready Logic : Subsystem
  ValidIn to Ready Logic1 : Subsystem
  y = u(2:end) : MATLAB Function  TreatAsAtomicUnit=on
  x' : Outport  VectorParamsAs1DForOutWhenUnconnected=off
  y' : Outport  Port=2  VectorParamsAs1DForOutWhenUnconnected=off
  u' : Outport  Port=3  VectorParamsAs1DForOutWhenUnconnected=off
  v' : Outport  Port=4  VectorParamsAs1DForOutWhenUnconnected=off
  validOut : Outport  Port=5  VectorParamsAs1DForOutWhenUnconnected=off
  validOut from rotate first element to real : Outport  Port=6  VectorParamsAs1DForOutWhenUnconnected=off
  ready : Outport  Port=7  VectorParamsAs1DForOutWhenUnconnected=off
  wires:
  QR 3rd and 4th Quadrant Compensation/1(x_out) -> Unit Delay Enabled Synchronous11/1
  QR 3rd and 4th Quadrant Compensation/3(u_out) -> Unit Delay Enabled Synchronous9/1
  QR 3rd and 4th Quadrant Compensation/2(y_out) -> Unit Delay Enabled Synchronous10/1
  QR 3rd and 4th Quadrant Compensation/4(v_out) -> Unit Delay Enabled Synchronous8/1
  Inverse CORDIC Gain3/1(Out1) -> Unit Delay Enabled Synchronous4/1
  Inverse CORDIC Gain4/1(Out1) -> Unit Delay Enabled Synchronous7/1
  x/1 -> Unit Delay Enabled Synchronous3/1
  Unit Delay Enabled Synchronous3/1 -> Rotate first element to real/1(x)
  u/1 -> Unit Delay Enabled Synchronous2/1
  v/1 -> Unit Delay Enabled Synchronous/1
  Inverse CORDIC Gain2/1(Out1) -> Unit Delay Enabled Synchronous5/1
  Unit Delay Enabled Synchronous11/1 -> "Q'B, R Row Rotations - Complex"/1(x)
  Unit Delay Enabled Synchronous10/1 -> "Q'B, R Row Rotations - Complex"/2(y)
  Unit Delay Enabled Synchronous9/1 -> "Q'B, R Row Rotations - Complex"/3(u)
  Unit Delay Enabled Synchronous8/1 -> "Q'B, R Row Rotations - Complex"/4(v)
  "Q'B, R Row Rotations - Complex"/1(x_out) -> Inverse CORDIC Gain4/1(In1)
  "Q'B, R Row Rotations - Complex"/3(u_out) -> Inverse CORDIC Gain2/1(In1)
  "Q'B, R Row Rotations - Complex"/4(v_out) -> Inverse CORDIC Gain3/1(In1)
  Inverse CORDIC Gain1/1(Out1) -> Unit Delay Enabled Synchronous6/1
  y = u(2:end)/1(y) -> y'/1
  Unit Delay Enabled Synchronous1/1 -> Rotate first element to real - 1/1(x)
  Unit Delay Enabled Synchronous/1 -> Rotate first element to real - 1/2(u)
  Rotate first element to real - 1/1(x') -> QR 3rd and 4th Quadrant Compensation/2(y)
  Rotate first element to real - 1/2(u') -> QR 3rd and 4th Quadrant Compensation/4(v)
  "Q'B, R Row Rotations - Complex"/2(y_out) -> Inverse CORDIC Gain1/1(In1)
  validIn/1 -> ValidIn to Ready Logic/2(validIn), Unit Delay Enabled Synchronous/2, Unit Delay Enabled Synchronous1/2, Unit Delay Enabled Synchronous2/2, Unit Delay Enabled Synchronous3/2, Delay11/1
  Delay11/1 -> ValidIn to Ready Logic1/2(validIn), Rotate first element to real/3(validIn), Rotate first element to real - 1/3(validIn)
  Rotate first element to real - 1/3(validOut) -> Unit Delay Enabled Synchronous8/2, Unit Delay Enabled Synchronous9/2, Unit Delay Enabled Synchronous10/2, Unit Delay Enabled Synchronous11/2, Delay12/1, validOut from rotate first element to real/1
  Unit Delay Enabled Synchronous7/1 -> x'/1
  Unit Delay Enabled Synchronous6/1 -> y = u(2:end)/1(u)
  Unit Delay Enabled Synchronous5/1 -> u'/1
  Unit Delay Enabled Synchronous4/1 -> v'/1
  Delay12/1 -> "Q'B, R Row Rotations - Complex"/5(validIn)
  "Q'B, R Row Rotations - Complex"/5(validOut) -> Delay17/1, Unit Delay Enabled Synchronous4/2, Unit Delay Enabled Synchronous5/2, Unit Delay Enabled Synchronous6/2, Unit Delay Enabled Synchronous7/2
  Delay17/1 -> validOut/1
  Rotate first element to real/4(ready) -> Terminator2/1
  Rotate first element to real/3(validOut) -> Terminator3/1
  Rotate first element to real/1(x') -> QR 3rd and 4th Quadrant Compensation/1(x)
  Rotate first element to real/2(u') -> QR 3rd and 4th Quadrant Compensation/3(u)
  Unit Delay Enabled Synchronous2/1 -> Rotate first element to real/2(u)
  y/1 -> Unit Delay Enabled Synchronous1/1
  ValidIn to Ready Logic/1(readyOut) -> ready/1
  ValidIn to Ready Logic1/1(readyOut) -> ValidIn to Ready Logic/1(readyIn)
  "Q'B, R Row Rotations - Complex"/6(ready) -> Terminator1/1
  Rotate first element to real - 1/4(ready) -> ValidIn to Ready Logic1/1(readyIn)

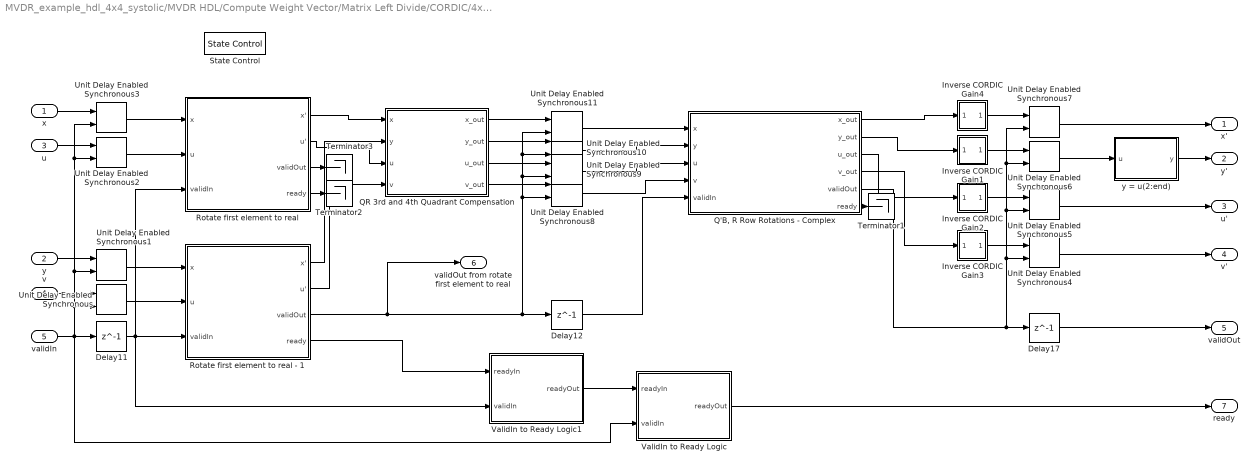
== system MVDR_example_hdl_4x4_systolic/MVDR HDL/Compute Weight Vector/Matrix Left Divide/CORDIC/4x4 Complex CORDIC Matrix Left Divide/Q'B, R 4x4 Complex CORDIC Systolic Array/Leading Complex Row Rotation - 4 ==
  x : Inport
  y : Inport  Port=2
  u : Inport  Port=3
  v : Inport  Port=4
  validIn : Inport  Port=5
  Delay11 : Delay  DelayLength=1
  Delay12 : Delay  DelayLength=1
  Delay17 : Delay  DelayLength=1
  Inverse CORDIC Gain1 : Subsystem  TreatAsAtomicUnit=on  mask{NumberOfCORDICIterations=NumberOfCORDICIterations}
      mask prompts: NumberOfCORDICIterations "Number of CORDIC Iterations"
      mask Display: disp('1/An')
  Inverse CORDIC Gain2 : Subsystem  TreatAsAtomicUnit=on  mask{NumberOfCORDICIterations=NumberOfCORDICIterations}
      mask prompts: NumberOfCORDICIterations "Number of CORDIC Iterations"
      mask Display: disp('1/An')
  Inverse CORDIC Gain3 : Subsystem  TreatAsAtomicUnit=on  mask{NumberOfCORDICIterations=NumberOfCORDICIterations}
      mask prompts: NumberOfCORDICIterations "Number of CORDIC Iterations"
      mask Display: disp('1/An')
  Inverse CORDIC Gain4 : Subsystem  TreatAsAtomicUnit=on  mask{NumberOfCORDICIterations=NumberOfCORDICIterations}
      mask prompts: NumberOfCORDICIterations "Number of CORDIC Iterations"
      mask Display: disp('1/An')
  "Q'B, R Row Rotations - Complex" : Subsystem  TreatAsAtomicUnit=on  mask{NumberOfCORDICIterations=NumberOfCORDICIterations}
      mask prompts: NumberOfCORDICIterations "Number of CORDIC Iterations"
  QR 3rd and 4th Quadrant Compensation : MATLAB Function  TreatAsAtomicUnit=on
  Rotate first element to real : Subsystem  TreatAsAtomicUnit=on  mask{NumberOfCORDICIterations=NumberOfCORDICIterations}
      mask prompts: NumberOfCORDICIterations "Number of CORDIC Iterations"
  Rotate first element to real - 1 : Subsystem  TreatAsAtomicUnit=on  mask{NumberOfCORDICIterations=NumberOfCORDICIterations}
      mask prompts: NumberOfCORDICIterations "Number of CORDIC Iterations"
  State Control : StateControl  StateControl=Synchronous
  Terminator1 : Terminator
  Terminator2 : Terminator
  Terminator3 : Terminator
  Unit Delay Enabled Synchronous{,1..11} (12 alike) : hdlsllib/Discrete/Unit Delay Enabled Synchronous  InitialCondition=0.0  SampleTime=-1
      settings: SourceProductBaseCode=SL
  ValidIn to Ready Logic : Subsystem
  ValidIn to Ready Logic1 : Subsystem
  y = u(2:end) : MATLAB Function  TreatAsAtomicUnit=on
  x' : Outport  VectorParamsAs1DForOutWhenUnconnected=off
  y' : Outport  Port=2  VectorParamsAs1DForOutWhenUnconnected=off
  u' : Outport  Port=3  VectorParamsAs1DForOutWhenUnconnected=off
  v' : Outport  Port=4  VectorParamsAs1DForOutWhenUnconnected=off
  validOut : Outport  Port=5  VectorParamsAs1DForOutWhenUnconnected=off
  validOut from rotate first element to real : Outport  Port=6  VectorParamsAs1DForOutWhenUnconnected=off
  ready : Outport  Port=7  VectorParamsAs1DForOutWhenUnconnected=off
  wires:
  QR 3rd and 4th Quadrant Compensation/1(x_out) -> Unit Delay Enabled Synchronous11/1
  QR 3rd and 4th Quadrant Compensation/3(u_out) -> Unit Delay Enabled Synchronous9/1
  QR 3rd and 4th Quadrant Compensation/2(y_out) -> Unit Delay Enabled Synchronous10/1
  QR 3rd and 4th Quadrant Compensation/4(v_out) -> Unit Delay Enabled Synchronous8/1
  Inverse CORDIC Gain3/1(Out1) -> Unit Delay Enabled Synchronous4/1
  Inverse CORDIC Gain4/1(Out1) -> Unit Delay Enabled Synchronous7/1
  x/1 -> Unit Delay Enabled Synchronous3/1
  Unit Delay Enabled Synchronous3/1 -> Rotate first element to real/1(x)
  u/1 -> Unit Delay Enabled Synchronous2/1
  v/1 -> Unit Delay Enabled Synchronous/1
  Inverse CORDIC Gain2/1(Out1) -> Unit Delay Enabled Synchronous5/1
  Unit Delay Enabled Synchronous11/1 -> "Q'B, R Row Rotations - Complex"/1(x)
  Unit Delay Enabled Synchronous10/1 -> "Q'B, R Row Rotations - Complex"/2(y)
  Unit Delay Enabled Synchronous9/1 -> "Q'B, R Row Rotations - Complex"/3(u)
  Unit Delay Enabled Synchronous8/1 -> "Q'B, R Row Rotations - Complex"/4(v)
  "Q'B, R Row Rotations - Complex"/1(x_out) -> Inverse CORDIC Gain4/1(In1)
  "Q'B, R Row Rotations - Complex"/3(u_out) -> Inverse CORDIC Gain2/1(In1)
  "Q'B, R Row Rotations - Complex"/4(v_out) -> Inverse CORDIC Gain3/1(In1)
  Inverse CORDIC Gain1/1(Out1) -> Unit Delay Enabled Synchronous6/1
  y = u(2:end)/1(y) -> y'/1
  Unit Delay Enabled Synchronous1/1 -> Rotate first element to real - 1/1(x)
  Unit Delay Enabled Synchronous/1 -> Rotate first element to real - 1/2(u)
  Rotate first element to real - 1/1(x') -> QR 3rd and 4th Quadrant Compensation/2(y)
  Rotate first element to real - 1/2(u') -> QR 3rd and 4th Quadrant Compensation/4(v)
  "Q'B, R Row Rotations - Complex"/2(y_out) -> Inverse CORDIC Gain1/1(In1)
  validIn/1 -> ValidIn to Ready Logic/2(validIn), Unit Delay Enabled Synchronous/2, Unit Delay Enabled Synchronous1/2, Unit Delay Enabled Synchronous2/2, Unit Delay Enabled Synchronous3/2, Delay11/1
  Delay11/1 -> ValidIn to Ready Logic1/2(validIn), Rotate first element to real/3(validIn), Rotate first element to real - 1/3(validIn)
  Rotate first element to real - 1/3(validOut) -> Unit Delay Enabled Synchronous8/2, Unit Delay Enabled Synchronous9/2, Unit Delay Enabled Synchronous10/2, Unit Delay Enabled Synchronous11/2, Delay12/1, validOut from rotate first element to real/1
  Unit Delay Enabled Synchronous7/1 -> x'/1
  Unit Delay Enabled Synchronous6/1 -> y = u(2:end)/1(u)
  Unit Delay Enabled Synchronous5/1 -> u'/1
  Unit Delay Enabled Synchronous4/1 -> v'/1
  Delay12/1 -> "Q'B, R Row Rotations - Complex"/5(validIn)
  "Q'B, R Row Rotations - Complex"/5(validOut) -> Delay17/1, Unit Delay Enabled Synchronous4/2, Unit Delay Enabled Synchronous5/2, Unit Delay Enabled Synchronous6/2, Unit Delay Enabled Synchronous7/2
  Delay17/1 -> validOut/1
  Rotate first element to real/4(ready) -> Terminator2/1
  Rotate first element to real/3(validOut) -> Terminator3/1
  Rotate first element to real/1(x') -> QR 3rd and 4th Quadrant Compensation/1(x)
  Rotate first element to real/2(u') -> QR 3rd and 4th Quadrant Compensation/3(u)
  Unit Delay Enabled Synchronous2/1 -> Rotate first element to real/2(u)
  y/1 -> Unit Delay Enabled Synchronous1/1
  ValidIn to Ready Logic/1(readyOut) -> ready/1
  ValidIn to Ready Logic1/1(readyOut) -> ValidIn to Ready Logic/1(readyIn)
  "Q'B, R Row Rotations - Complex"/6(ready) -> Terminator1/1
  Rotate first element to real - 1/4(ready) -> ValidIn to Ready Logic1/1(readyIn)

== system MVDR_example_hdl_4x4_systolic/MVDR HDL/Compute Weight Vector/Matrix Left Divide/CORDIC/4x4 Complex CORDIC Matrix Left Divide/Q'B, R 4x4 Complex CORDIC Systolic Array/Rotate first element to real ==
  x : Inport
  u : Inport  Port=2
  validIn : Inport  Port=3
  Complex to Real-Imag : ComplexToRealImag
  Complex to Real-Imag1 : ComplexToRealImag
  Delay{4..7,9..10,15} (7 alike) : Delay  DelayLength=1
  Force imaginary part to exactly zero : MATLAB Function  TreatAsAtomicUnit=on
  Inverse CORDIC Gain1 : Subsystem  TreatAsAtomicUnit=on  mask{NumberOfCORDICIterations=NumberOfCORDICIterations}
      mask prompts: NumberOfCORDICIterations "Number of CORDIC Iterations"
      mask Display: disp('1/An')
  Inverse CORDIC Gain2 : Subsystem  TreatAsAtomicUnit=on  mask{NumberOfCORDICIterations=NumberOfCORDICIterations}
      mask prompts: NumberOfCORDICIterations "Number of CORDIC Iterations"
      mask Display: disp('1/An')
  Inverse CORDIC Gain3 : Subsystem  TreatAsAtomicUnit=on  mask{NumberOfCORDICIterations=NumberOfCORDICIterations}
      mask prompts: NumberOfCORDICIterations "Number of CORDIC Iterations"
      mask Display: disp('1/An')
  Inverse CORDIC Gain4 : Subsystem  TreatAsAtomicUnit=on  mask{NumberOfCORDICIterations=NumberOfCORDICIterations}
      mask prompts: NumberOfCORDICIterations "Number of CORDIC Iterations"
      mask Display: disp('1/An')
  "Q'B, R Row Rotations - Real" : Subsystem  TreatAsAtomicUnit=on  mask{NumberOfCORDICIterations=NumberOfCORDICIterations}
      mask prompts: NumberOfCORDICIterations "Number of CORDIC Iterations"
  QR 3rd and 4th Quadrant Compensation : MATLAB Function  TreatAsAtomicUnit=on
  Real-Imag to Complex : RealImagToComplex
  Real-Imag to Complex1 : RealImagToComplex
  State Control : StateControl  StateControl=Synchronous
  Unit Delay Enabled Synchronous{,1..3} (4 alike) : hdlsllib/Discrete/Unit Delay Enabled Synchronous  InitialCondition=0.0  SampleTime=-1
      settings: SourceProductBaseCode=SL
  ValidIn to Ready Logic with Delay : Subsystem
  x' : Outport  VectorParamsAs1DForOutWhenUnconnected=off
  u' : Outport  Port=2  VectorParamsAs1DForOutWhenUnconnected=off
  validOut : Outport  Port=3  VectorParamsAs1DForOutWhenUnconnected=off
  ready : Outport  Port=4  VectorParamsAs1DForOutWhenUnconnected=off
  wires:
  QR 3rd and 4th Quadrant Compensation/1(x_out) -> Delay4/1
  QR 3rd and 4th Quadrant Compensation/3(u_out) -> Delay6/1
  QR 3rd and 4th Quadrant Compensation/2(y_out) -> Delay5/1
  QR 3rd and 4th Quadrant Compensation/4(v_out) -> Delay7/1
  Complex to Real-Imag/1 -> QR 3rd and 4th Quadrant Compensation/1(x)
  Complex to Real-Imag/2 -> QR 3rd and 4th Quadrant Compensation/2(y)
  Complex to Real-Imag1/1 -> QR 3rd and 4th Quadrant Compensation/3(u)
  Complex to Real-Imag1/2 -> QR 3rd and 4th Quadrant Compensation/4(v)
  Delay4/1 -> "Q'B, R Row Rotations - Real"/1(x)
  Delay5/1 -> "Q'B, R Row Rotations - Real"/2(y)
  Delay6/1 -> "Q'B, R Row Rotations - Real"/3(u)
  Delay7/1 -> "Q'B, R Row Rotations - Real"/4(v)
  "Q'B, R Row Rotations - Real"/1(x_out) -> Inverse CORDIC Gain4/1(In1)
  "Q'B, R Row Rotations - Real"/3(u_out) -> Inverse CORDIC Gain2/1(In1)
  "Q'B, R Row Rotations - Real"/4(v_out) -> Inverse CORDIC Gain3/1(In1)
  x/1 -> Unit Delay Enabled Synchronous1/1
  u/1 -> Unit Delay Enabled Synchronous/1
  "Q'B, R Row Rotations - Real"/2(y_out) -> Inverse CORDIC Gain1/1(In1)
  Force imaginary part to exactly zero/1(y) -> Real-Imag to Complex/2
  Delay9/1 -> ValidIn to Ready Logic with Delay/3(validIn), Delay10/1
  validIn/1 -> Unit Delay Enabled Synchronous/2, Unit Delay Enabled Synchronous1/2, Delay9/1
  Delay10/1 -> ValidIn to Ready Logic with Delay/2(validIn * z^-1), "Q'B, R Row Rotations - Real"/5(validIn)
  Inverse CORDIC Gain4/1(Out1) -> Real-Imag to Complex/1
  Inverse CORDIC Gain1/1(Out1) -> Force imaginary part to exactly zero/1(u)
  Inverse CORDIC Gain2/1(Out1) -> Real-Imag to Complex1/1
  Inverse CORDIC Gain3/1(Out1) -> Real-Imag to Complex1/2
  "Q'B, R Row Rotations - Real"/5(validOut) -> Unit Delay Enabled Synchronous2/2, Unit Delay Enabled Synchronous3/2, Delay15/1
  Delay15/1 -> validOut/1
  ValidIn to Ready Logic with Delay/1(readyOut) -> ready/1
  "Q'B, R Row Rotations - Real"/6(ready) -> ValidIn to Ready Logic with Delay/1(readyIn)
  Unit Delay Enabled Synchronous/1 -> Complex to Real-Imag1/1
  Unit Delay Enabled Synchronous1/1 -> Complex to Real-Imag/1
  Real-Imag to Complex1/1 -> Unit Delay Enabled Synchronous2/1
  Unit Delay Enabled Synchronous2/1 -> u'/1
  Real-Imag to Complex/1 -> Unit Delay Enabled Synchronous3/1
  Unit Delay Enabled Synchronous3/1 -> x'/1

== system MVDR_example_hdl_4x4_systolic/MVDR HDL/Compute Weight Vector/Matrix Left Divide/CORDIC/4x4 Complex CORDIC Matrix Left Divide/Q'B, R 4x4 Complex CORDIC Systolic Array/ValidIn to Ready Logic with Delay ==
  readyIn : Inport
  validIn * z^-1 : Inport  Port=2
  validIn : Inport  Port=3
  AND : Logic  IconShape=distinctive  AllPortsSameDT=off  OutDataTypeStr=boolean
  AND1 : Logic  IconShape=distinctive  AllPortsSameDT=off  OutDataTypeStr=boolean
  NOT : Logic  Operator=NOT  IconShape=distinctive  AllPortsSameDT=off  OutDataTypeStr=boolean
  NOT1 : Logic  Operator=NOT  IconShape=distinctive  AllPortsSameDT=off  OutDataTypeStr=boolean
  readyOut : Outport  VectorParamsAs1DForOutWhenUnconnected=off
  wires:
  validIn * z^-1/1 -> NOT/1
  validIn/1 -> NOT1/1
  readyIn/1 -> AND/1
  AND1/1 -> readyOut/1
  NOT1/1 -> AND1/2
  NOT/1 -> AND/2
  AND/1 -> AND1/1

== system MVDR_example_hdl_4x4_systolic/MVDR HDL/Compute Weight Vector/Matrix Left Divide/CORDIC/4x4 Complex CORDIC Matrix Left Divide/Back Substitute 4x4 Complex CORDIC/Invert first element - Folded/CORDIC Reciprocal Normalized, Folded ==
  x : Inport
  validIn : Inport  Port=2
  CORDIC Reciprocal Rotations- Folded : Subsystem  TreatAsAtomicUnit=on  mask{NumberOfCORDICIterations=NumberOfCORDICIterations}
      mask prompts: NumberOfCORDICIterations "Number of CORDIC Iterations"
  Change sign : MATLAB Function  TreatAsAtomicUnit=on
  Delay{,1..3,5,10} (6 alike) : Delay  DelayLength=1
  Normalizer : Subsystem
  State Control : StateControl  StateControl=Synchronous
  Unit Delay Enabled Synchronous : hdlsllib/Discrete/Unit Delay Enabled Synchronous  InitialCondition=0.0  SampleTime=-1
      settings: SourceProductBaseCode=SL
  Unit Delay Enabled Synchronous1 : hdlsllib/Discrete/Unit Delay Enabled Synchronous  InitialCondition=0.0  SampleTime=-1
      settings: SourceProductBaseCode=SL
  ValidIn to Ready Logic : Subsystem
  ValidIn to Ready Logic1 : Subsystem
  ValidIn to Ready Logic2 : Subsystem
  1/x_normalized : Outport  VectorParamsAs1DForOutWhenUnconnected=off
  shift_value : Outport  Port=2  VectorParamsAs1DForOutWhenUnconnected=off
  validOut : Outport  Port=3  VectorParamsAs1DForOutWhenUnconnected=off
  ready : Outport  Port=4  VectorParamsAs1DForOutWhenUnconnected=off
  wires:
  Unit Delay Enabled Synchronous/1 -> Normalizer/1(u)
  Normalizer/1(u_normalized) -> Delay/1
  Change sign/1(y) -> Delay3/1
  Unit Delay Enabled Synchronous1/1 -> Delay5/1
  Delay3/1 -> 1/x_normalized/1
  Normalizer/2(is_negative) -> Change sign/2(is_negative)
  Delay5/1 -> shift_value/1
  CORDIC Reciprocal Rotations- Folded/1(z_out) -> Change sign/1(x)
  Normalizer/3(shift_amount) -> Unit Delay Enabled Synchronous1/1
  x/1 -> Unit Delay Enabled Synchronous/1
  Delay/1 -> CORDIC Reciprocal Rotations- Folded/1(x_in)
  Normalizer/4(validOut) -> ValidIn to Ready Logic1/2(validIn), Delay1/1, Unit Delay Enabled Synchronous1/2
  validIn/1 -> Unit Delay Enabled Synchronous/2, Delay10/1
  Delay10/1 -> ValidIn to Ready Logic2/2(validIn), Normalizer/2(validIn)
  CORDIC Reciprocal Rotations- Folded/3(ready) -> ValidIn to Ready Logic/1(readyIn)
  ValidIn to Ready Logic/1(readyOut) -> ValidIn to Ready Logic1/1(readyIn)
  ValidIn to Ready Logic1/1(readyOut) -> ValidIn to Ready Logic2/1(readyIn)
  ValidIn to Ready Logic2/1(readyOut) -> ready/1
  CORDIC Reciprocal Rotations- Folded/2(validOut) -> Delay2/1
  Delay2/1 -> validOut/1
  Delay1/1 -> CORDIC Reciprocal Rotations- Folded/2(validIn), ValidIn to Ready Logic/2(validIn)

== system MVDR_example_hdl_4x4_systolic/MVDR HDL/Compute Weight Vector/Matrix Left Divide/CORDIC/4x4 Complex CORDIC Matrix Left Divide/Back Substitute 4x4 Complex CORDIC/Invert first element - Folded/ValidIn to Ready Logic ==
  readyIn : Inport
  validIn : Inport  Port=2
  AND : Logic  IconShape=distinctive  AllPortsSameDT=off  OutDataTypeStr=boolean
  NOT : Logic  Operator=NOT  IconShape=distinctive  AllPortsSameDT=off  OutDataTypeStr=boolean
  readyOut : Outport  VectorParamsAs1DForOutWhenUnconnected=off
  wires:
  validIn/1 -> NOT/1
  readyIn/1 -> AND/1
  AND/1 -> readyOut/1
  NOT/1 -> AND/2

== system MVDR_example_hdl_4x4_systolic/MVDR HDL/Compute Weight Vector/Matrix Left Divide/CORDIC/4x4 Complex CORDIC Matrix Left Divide/Back Substitute 4x4 Complex CORDIC/Invert first element - Folded1/CORDIC Reciprocal Normalized, Folded ==
  x : Inport
  validIn : Inport  Port=2
  CORDIC Reciprocal Rotations- Folded : Subsystem  TreatAsAtomicUnit=on  mask{NumberOfCORDICIterations=NumberOfCORDICIterations}
      mask prompts: NumberOfCORDICIterations "Number of CORDIC Iterations"
  Change sign : MATLAB Function  TreatAsAtomicUnit=on
  Delay{,1..3,5,10} (6 alike) : Delay  DelayLength=1
  Normalizer : Subsystem
  State Control : StateControl  StateControl=Synchronous
  Unit Delay Enabled Synchronous : hdlsllib/Discrete/Unit Delay Enabled Synchronous  InitialCondition=0.0  SampleTime=-1
      settings: SourceProductBaseCode=SL
  Unit Delay Enabled Synchronous1 : hdlsllib/Discrete/Unit Delay Enabled Synchronous  InitialCondition=0.0  SampleTime=-1
      settings: SourceProductBaseCode=SL
  ValidIn to Ready Logic : Subsystem
  ValidIn to Ready Logic1 : Subsystem
  ValidIn to Ready Logic2 : Subsystem
  1/x_normalized : Outport  VectorParamsAs1DForOutWhenUnconnected=off
  shift_value : Outport  Port=2  VectorParamsAs1DForOutWhenUnconnected=off
  validOut : Outport  Port=3  VectorParamsAs1DForOutWhenUnconnected=off
  ready : Outport  Port=4  VectorParamsAs1DForOutWhenUnconnected=off
  wires:
  Delay1/1 -> ValidIn to Ready Logic/2(validIn), CORDIC Reciprocal Rotations- Folded/2(validIn)
  Delay2/1 -> validOut/1
  CORDIC Reciprocal Rotations- Folded/2(validOut) -> Delay2/1
  ValidIn to Ready Logic2/1(readyOut) -> ready/1
  ValidIn to Ready Logic1/1(readyOut) -> ValidIn to Ready Logic2/1(readyIn)
  ValidIn to Ready Logic/1(readyOut) -> ValidIn to Ready Logic1/1(readyIn)
  CORDIC Reciprocal Rotations- Folded/3(ready) -> ValidIn to Ready Logic/1(readyIn)
  Delay10/1 -> Normalizer/2(validIn), ValidIn to Ready Logic2/2(validIn)
  validIn/1 -> Delay10/1, Unit Delay Enabled Synchronous/2
  Normalizer/4(validOut) -> Unit Delay Enabled Synchronous1/2, Delay1/1, ValidIn to Ready Logic1/2(validIn)
  Delay/1 -> CORDIC Reciprocal Rotations- Folded/1(x_in)
  x/1 -> Unit Delay Enabled Synchronous/1
  Normalizer/3(shift_amount) -> Unit Delay Enabled Synchronous1/1
  CORDIC Reciprocal Rotations- Folded/1(z_out) -> Change sign/1(x)
  Delay5/1 -> shift_value/1
  Normalizer/2(is_negative) -> Change sign/2(is_negative)
  Delay3/1 -> 1/x_normalized/1
  Unit Delay Enabled Synchronous1/1 -> Delay5/1
  Change sign/1(y) -> Delay3/1
  Normalizer/1(u_normalized) -> Delay/1
  Unit Delay Enabled Synchronous/1 -> Normalizer/1(u)
